simulink model "off_grid_solar_pv"  (R2016a)
settings: Solver=ode23t  SolverMode=SingleTasking  StartTime=0.0  StopTime=0.1  RelTol=1e-3
undefined symbols (not defined in the file): Acid, Lead
libraries: spsIGBTDiodeLib x4, spsSeriesRLCBranchLib x3, spsVoltageMeasurementLib x2, spsBatteryLib x1, spsDiodeLib x1, mqtt x1, spsMosfetLib x1, spsPVArrayLib x1, simulink x1, spsSeriesRLCLoadLib x1, spsVariableRatioTransformerLib x1, spspowerguiLib x1
settings Model: Creator=ISURU LOLLA  LastModifiedBy=ISURU LOLLA
settings DataIOCC: ReturnWorkspaceOutputs=on
settings DebuggingCC: SFUnexpectedBacktrackingDiag=error  SFNoUnconditionalDefaultTransitionDiag=error
settings SFSimCC: SimUseLocalCustomCode=on
settings RTWCC: RTWUseLocalCustomCode=on
settings GRTTargetCC: TargetLangStandard=C99 (ISO)
settings ConfigComp: CovMetricSettings=dwe  CovSaveCumulativeToWorkspaceVar=off  CovSaveSingleToWorkspaceVar=off  CovExternalEMLEnable=on

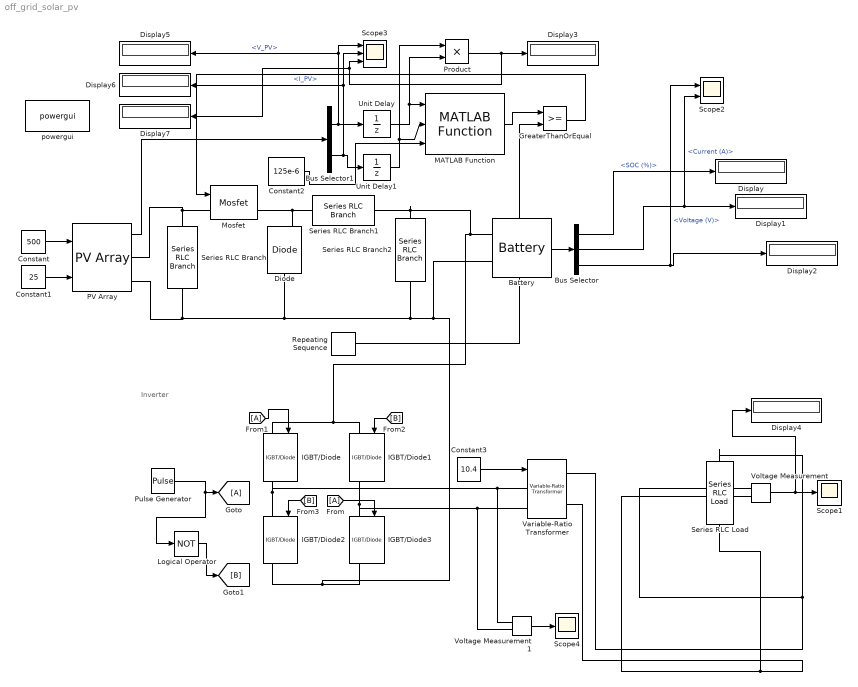
== system off_grid_solar_pv ==
  note: Inverter
  Battery : spsBatteryLib/Battery  BatType=Lead-Acid  ShowTempParam=off  ThermalPreset=no  ShowAgeParam=off  NomV=24  NomQ=317.5  SOC=20  Batt_Tr=1  PresetModel=on  MaxQ=330.7292  MinV=18  FullV=26.1316  Dis_rate=63.5  R=0.00075591  Normal_OP=98.5132  expZone="[24.4342      1.05833]"  current=[6.5 13 32.5]  Units=Time  Tci=20  NomT=20  T2=-30  MaxQ2=4.8  FullV2=7.1  Normal_OP2=5.655  expZone2="[6.58           1]"  Rca=0.6  ti=2000  Dp=0  Neq0=0  Tsim=1e6  Ta1=25  Qeol=5.4*0.9  Reol=0.013333*1.2  Char_age=[2.3478, 3]  Dis_age=[2.3478, 10]  N1=1500  N2=10500  N3=1000  N4=1400  Ta2=45  N5=950
  Bus Selector : BusSelector  OutputSignals=SOC (%),Current (A),Voltage (V)
  Bus Selector1 : BusSelector  OutputSignals=V_PV,I_PV
  Constant : Constant  Value=500
  Constant1 : Constant  Value=25
  Constant2 : Constant  Value=125e-6
  Constant3 : Constant  Value=10.4
  Diode : spsDiodeLib/Diode  Ron=0.001  Lon=0  Vf=0.8  IC=0  UseSnubber=0  Rs=500  Cs=250e-9  Measurements=on
  Display{,1..7} (8 alike) : Display
  GreaterThanOrEqual : RelationalOperator  OutDataTypeStr=boolean
  IGBT/Diode{,1..3} (4 alike) : spsIGBTDiodeLib/IGBT//Diode  Ron=1e-3  Rs=1e5  Cs=inf  Measurements=on
  Logical Operator : Logic  Operator=NOT  AllPortsSameDT=off  OutDataTypeStr=boolean
  MATLAB Function : mqtt/MATLAB Function  SystemSampleTime=-1  Latency=0  AutoFrameSizeCalculation=off
  Mosfet : spsMosfetLib/Mosfet  Ron=0.1  Lon=0  Rd=0.01  Vfd=0  IC=0  Rs=1e5  Cs=inf  Measurements=on
  PV Array : spsPVArrayLib/PV Array  Npar=1  Nser=2  PlotType=array @ 25 deg.C & specified irradiances  S_vec="[ 1000  500  100 ]"  Temp_C_vec="[ 45 25  ]"  ModuleName=A10Green Technology A10J-S72-175  PlotWhenSelected=off  Pm=175.0914  Ncell=72  Voc=43.99  Isc=5.17  Vm=36.63  Im=4.78  beta_Voc_pc=-0.3616  alpha_Isc_pc=0.041509  beta_Voc=-0.15907  alpha_Isc=0.002146  IL=5.178  I0=1.7842e-10  nI=0.98852  Rsh=249.6758  Rs=0.38412  RobustModel=off  RobustCellTemperature=313.3991  BAL=on  Tc=1e-6  Tfilter=5e-5
  Product : Product
  Pulse Generator : DiscretePulseGenerator  PulseType=Time based  Period=0.02  PulseWidth=50
  Repeating Sequence : simulink/Sources/Repeating Sequence  rep_seq_t=[0 0.0002]  rep_seq_y=[0 1]
  Scope1 : Scope
  Scope2 : Scope  NumInputPorts=2
  Scope3 : Scope  NumInputPorts=3
  Scope4 : Scope
  Series RLC Branch : spsSeriesRLCBranchLib/Series RLC Branch  LConnTagsString=__new0  RConnTagsString=__new0  BranchType=RC  Resistance=0.0001  Inductance=1e-3  SetiL0=off  InitialCurrent=0  Capacitance=1000e-6  Setx0=off  InitialVoltage=0  Measurements=None
  Series RLC Branch1 : spsSeriesRLCBranchLib/Series RLC Branch  LConnTagsString=__new0  RConnTagsString=__new0  BranchType=L  Resistance=1  Inductance=0.783e-3  SetiL0=off  InitialCurrent=0  Capacitance=1e-6  Setx0=off  InitialVoltage=0  Measurements=None
  Series RLC Branch2 : spsSeriesRLCBranchLib/Series RLC Branch  LConnTagsString=__new0  RConnTagsString=__new0  BranchType=C  Resistance=1  Inductance=0.783e-3  SetiL0=off  InitialCurrent=0  Capacitance=364e-6  Setx0=off  InitialVoltage=0  Measurements=None
  Series RLC Load : spsSeriesRLCLoadLib/Series RLC Load  LConnTagsString=a  RConnTagsString=__new0  NominalVoltage=230  NominalFrequency=50  ActivePower=1000  InductivePower=0  CapacitivePower=0  Setx0=off  InitialVoltage=0  SetiL0=off  InitialCurrent=0  Measurements=None  LoadType=constant Z
  Unit Delay : UnitDelay  SampleTime=1e-4  HasFrameUpgradeWarning=on
  Unit Delay1 : UnitDelay  SampleTime=1e-4  HasFrameUpgradeWarning=on
  Variable-Ratio Transformer : spsVariableRatioTransformerLib/Variable-Ratio Transformer
  Voltage Measurement : spsVoltageMeasurementLib/Voltage Measurement  PhasorSimulation=off  OutputType=Complex  PSBequivalent=0
  Voltage Measurement1 : spsVoltageMeasurementLib/Voltage Measurement  PhasorSimulation=off  OutputType=Complex  PSBequivalent=0
  powergui : spspowerguiLib/powergui  Priority=1  SimulationMode=Discrete  SampleTime=1e-6  frequency=60  Iterations=50  frequencyindice=0  Pbase=100e6  ErrMax=1e-4  UnitsV=kV  UnitsW=MW  buscounter=0  FunctionMessages=off  echomessages=off  EnableUseOfTLC=off  CurrentSourceSwitches=off  DisableSnubberDevices=off  DisableRonSwitches=off  DisableVfSwitches=off  DisplayEquations=off  AutomaticDiscreteSolvers=off  SolverType=Tustin/Backward Euler (TBE)  Interpol=off  ExternalGateDelay=off  methode=off  Ts=100  x0status=blocks  SPID=on  SwTol=0  HookPort=off  NonlinearTolerance=1e-4  nMaxIteration=100  ContinueOnMaxIteration=off  RestoreLinks=warning  ResistiveCurrentMeasurement=off  Frange=[0:2:500]  Ylog=off  Xlog=on  ShowGrid=off  save=off  variable=ZData  structure=0  ZoomFFT=off  StartTime=0.0  cycles=1  DisplayStyle=1  fundamental=60  FreqAxis=off  MaxFrequency=1000  frequencyindicesteady=1  RmsSteady=1  display=off
  wires:
  Constant/1 -> PV Array/1
  Constant1/1 -> PV Array/2
  Battery/1 -> Bus Selector/1
  Bus Selector/1 -> Display/1  "<SOC (%)>"
  Bus Selector/2 -> Scope2/2, Display1/1  "<Current (A)>"
  Bus Selector/3 -> Scope2/1, Display2/1  "<Voltage (V)>"
  PV Array/1 -> Bus Selector1/1
  Bus Selector1/1 -> Display5/1, Scope3/1, Unit Delay/1  "<V_PV>"
  Bus Selector1/2 -> Display6/1, Scope3/2, Unit Delay1/1  "<I_PV>"
  Unit Delay/1 -> MATLAB Function/1, Product/2
  Unit Delay1/1 -> MATLAB Function/2, Product/1
  GreaterThanOrEqual/1 -> Mosfet/1
  Repeating Sequence/1 -> GreaterThanOrEqual/2
  Product/1 -> Display7/1, Scope3/3, Display3/1
  Constant2/1 -> MATLAB Function/3
  MATLAB Function/1 -> GreaterThanOrEqual/1
  Logical Operator/1 -> [B]
  [A] -> IGBT/Diode/1
  [B] -> IGBT/Diode2/1
  Constant3/1 -> Variable-Ratio Transformer/1
  Voltage Measurement/1 -> Display4/1, Scope1/1
  [A] -> IGBT/Diode3/1
  Pulse Generator/1 -> Logical Operator/1, [A]
  [B] -> IGBT/Diode1/1
  Voltage Measurement1/1 -> Scope4/1
  connections:
  Series RLC Branch/LConn1 -- Mosfet/LConn1 -- PV Array/RConn1
  IGBT/Diode3/RConn1 -- Battery/LConn2 -- Series RLC Branch2/RConn1 -- Series RLC Branch/RConn1 -- PV Array/RConn2 -- Diode/LConn1 -- IGBT/Diode2/RConn1
  Mosfet/RConn1 -- Series RLC Branch1/LConn1 -- Diode/RConn1
  Variable-Ratio Transformer/LConn2 -- Voltage Measurement1/LConn2 -- IGBT/Diode3/LConn1 -- IGBT/Diode1/RConn1
  IGBT/Diode/RConn1 -- IGBT/Diode2/LConn1 -- Voltage Measurement1/LConn1 -- Variable-Ratio Transformer/LConn1
  Voltage Measurement/LConn2 -- Variable-Ratio Transformer/RConn2 -- Series RLC Load/RConn1
  Series RLC Load/LConn1 -- Variable-Ratio Transformer/RConn1 -- Voltage Measurement/LConn1
  Series RLC Branch1/RConn1 -- IGBT/Diode1/LConn1 -- IGBT/Diode/LConn1 -- Battery/LConn1 -- Series RLC Branch2/LConn1
